simulink model "I2cTempSensor"  (R2018b)
settings: Solver=VariableStepAuto  StartTime=0.0  StopTime=10.0  RelTol=1e-3
libraries: arduinolib x1
settings Model: Creator=apple  LastModifiedBy=apple

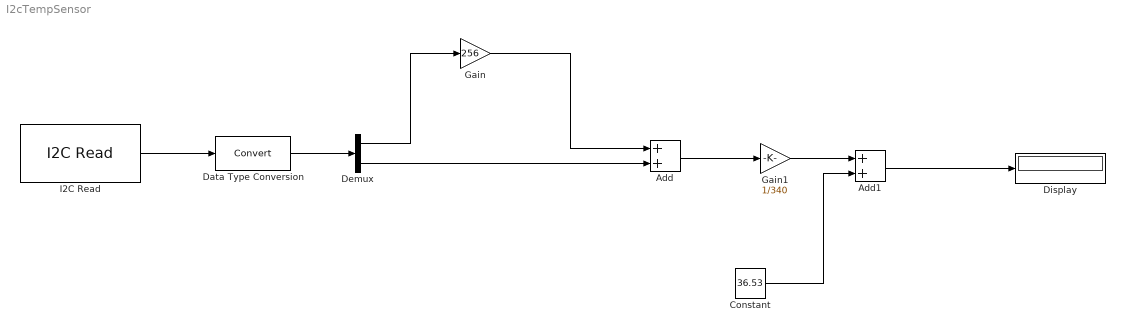
== system I2cTempSensor ==
  Add : Sum
  Add1 : Sum
  Constant : Constant  Value=36.53
  Data Type Conversion : DataTypeConversion
  Demux : Demux  Outputs=2
  Display : Display
  Gain : Gain  Gain=256
  Gain1 : Gain  Gain=1/340
  I2C Read : arduinolib/I2C Read  I2CModule=0  Mode=Master  SlaveAddress=104  SlaveByteOrder=BigEndian  Direction=Receiver  RegisterAddressMode=on  RegisterAddress=65  SlaveDataType=uint8  DataLength=2  NoAck=off  RepeatedStart=off  OutputStatus=off  blockPlatform=ARDUINO  SampleTime=0.1
      settings: SourceProductName=Simulink Support Package for Arduino Hardware  SourceProductBaseCode=ARDUINO
  wires:
  I2C Read/1 -> Data Type Conversion/1
  Data Type Conversion/1 -> Demux/1
  Demux/1 -> Gain/1
  Demux/2 -> Add/2
  Gain/1 -> Add/1
  Add/1 -> Gain1/1
  Gain1/1 -> Add1/1
  Constant/1 -> Add1/2
  Add1/1 -> Display/1
